simulink model "model_main4"  (R2023b)
settings: Solver=ode4  StartTime=0.0  StopTime=1000  FixedStep=dt  RelTol=1e-3
values from neighbouring files (symbols this model uses):
  dt = 0.01    [model_init.m]
  Iws = diag([1 1 1 1])*0.227    [model_init.m]
  m_tot = 3019.19    [model_init.m]
  Omega1_init = 1000*rpm2rad    (= 104.71975512)    [model_init.m]
  Omega2_init = 1000*rpm2rad    (= 104.71975512)    [model_init.m]
  Omega3_init = 1000*rpm2rad    (= 104.71975512)    [model_init.m]
  Omega4_init = 1000*rpm2rad    (= 104.71975512)    [model_init.m]
  qb0 = eul2quat(ag0','ZYX')'    [model_init.m]
  rad2rpm = 1/rpm2rad    (= 9.54929658551)    [model_init.m]
  RCS_F = 1.0    (= 1)    [model_init.m]
  RCS_Pos = [RCS1_POS , RCS2_POS , RCS3_POS , RCS4_POS ,            RCS5_POS , RCS6_POS , RCS7_POS , RCS8_POS ,            RCS9_POS , RCS10_POS, RCS11_POS, RCS12_POS,            RCS13_POS, RCS14_POS, RCS15_POS, RCS16_POS]    [model_init.m]
  RCS_PWM_Freq = 0.5    [model_init.m]
  RCS_Sampling_time = 0.01    [model_init.m]
  RCS_THR_vec = [RCS1_THR , RCS2_THR , RCS3_THR , RCS4_THR,                 RCS5_THR , RCS6_THR , RCS7_THR , RCS8_THR,                 RCS9_THR , RCS10_THR, RCS11_THR, RCS12_THR,                 RCS13_THR, RCS14_THR, RCS15_THR, RCS16_THR]    [model_init.m]
  REL_TS_POS_I_0 = TS_pos0 - SC_pos0    [model_init.m]
  REL_TS_VEL_I_0 = TS_vel0 - SC_vel0    [model_init.m]
  RW_As = [RW1_Axis,RW2_Axis,RW3_Axis,RW4_Axis]    [model_init.m]
  RW_Omegad_max = 4200*rpm2rad    (= 439.822971503)    [model_init.m]
  SC_Ib = [1257.52 -0.07285  -0.0345 ... (first row only)    [model_init.m]
  SC_state0 = kepel_statvec (SC_Kepler)    [model_init.m]
  TS_Ib = diag([1 1 1])    [model_init.m]
  TS_qb0 = angle2quat(deg2rad(0),deg2rad(0),deg2rad(0),'ZYX')'    [model_init.m]
  TS_state0 = kepel_statvec (TS_Kepler)    [model_init.m]
  TS_wb0 = deg2rad([0 0 0]')    [model_init.m]
  wb0 = [0 0 0]'    [model_init.m]
undefined symbols (not defined in the file or in its folder): norm_Ib, RCS_F_vec, RCS_pos, RW_Max_Speed, SS_Total_Mass, TC_Kepler
libraries: simulink x16, simulink_extras x13, sharedtransform x9, aerolibutil x8
(part 2 of 2)

== matlab function model_main4/Subsystem/Attitude_PD_control1 ==
  settings: updateMethod=DISCRETE
  data: F_B_cmd output; r_I input; v_I input; q_IB input; r_d input; v_d input; a_d input; m input
function F_B_cmd  = CTRL_WRENCH_6DOF(r_I, v_I, q_IB, r_d, v_d, a_d, m)
%#codegen
% ============================================================
% Controller block
% Input :
%   r_I      [3x1] current position in inertial frame
%   v_I      [3x1] current velocity in inertial frame
%   q_IB     [4x1] quaternion [qw qx qy qz], Body -> Inertial
%   omega_B  [3x1] current angular velocity in body frame
%
%   r_d      [3x1] desired position in inertial frame
%   v_d      [3x1] desired velocity in inertial frame
%   a_d      [3x1] desired acceleration in inertial frame
%   q_d      [4x1] desired quaternion, Body -> Inertial
%   omega_d_B[3x1] desired angular velocity in body frame
%
%   m        scalar mass
%   J        [3x3] inertia matrix in body frame
%
% Output:
%   F_B_cmd    [3x1] desired total body force
%   tau_B_cmd  [3x1] desired total body torque
% ============================================================

    % -------------------------
    % Quaternion normalize
    % -------------------------
    q_IB = quat_normalize(q_IB); 

    % -------------------------
    % Gains (example)
    % -------------------------
    Kp_r = 10*diag([0.01, 0.006, 0.006]);   % position gain
    Kd_r = 100*diag([0.01, 0.01, 0.01]);   % velocity damping
 
    % Kp_r = diag([0.010, 0.010, 0.010]);   % position gain
    % Kd_r = diag([0.060, 0.060, 0.060]);   % velocity damping

    % -------------------------
    % Position control
    % inertial acceleration command
    % -------------------------
    e_r = r_I - r_d;
    e_v = v_I - v_d;

    a_cmd   = a_d - Kp_r * e_r - Kd_r * e_v;
    F_I_cmd = m * a_cmd;

    % Convert inertial force -> body force
    R_IB    = quat_to_rotm(q_IB);
    F_B_cmd = R_IB.' * F_I_cmd;
 
end


% ============================================================
% Local helper functions
% ============================================================

function qn = quat_normalize(q)
    n = norm(q);
    if n < 1e-12
        qn = [1;0;0;0];
    else
        qn = q / n;
    end
end
 

function R = quat_to_rotm(q)
    % q = [qw qx qy qz], Body -> Inertial
    qw = q(1); qx = q(2); qy = q(3); qz = q(4);

    R = [1-2*(qy^2+qz^2),   2*(qx*qy-qz*qw),   2*(qx*qz+qy*qw);
         2*(qx*qy+qz*qw),   1-2*(qx^2+qz^2),   2*(qy*qz-qx*qw);
         2*(qx*qz-qy*qw),   2*(qy*qz+qx*qw),   1-2*(qx^2+qy^2)];
end

== matlab function model_main4/Subsystem/Thruster Allocation ==
  settings: updateMethod=DISCRETE
  data: u_pwm output; F_B_cmd input; tau_B_cmd input; F_B_real output; tau_B_real output; r input; d input; F_max input
function [u_pwm, F_B_real, tau_B_real] = ALLOC_THRUSTER_PWM_16(F_B_cmd, tau_B_cmd, r, d, F_max)
%#codegen
% ============================================================
% Allocation block
% Input :
%   F_B_cmd    [3x1] desired total body force
%   tau_B_cmd  [3x1] desired total body torque
%
% Output:
%   u_pwm      [12x1] thruster duty command, 0 ~ 1
%   F_B_real   [3x1] realized body force after allocation
%   tau_B_real [3x1] realized body torque after allocation
%
% Example:
%   12-thruster layout for 6DoF control
%   Replace thruster geometry / Tmax below with your real spacecraft values.
% ============================================================

    % Build 6x12 thruster mapping matrix A
    A = build_thruster_matrix( 16, r, d, F_max);

    % Desired wrench
    w_cmd = [F_B_cmd; tau_B_cmd];

    % Bounded least-squares allocation: 0 <= u <= 1
    u_pwm = bounded_allocator_0_1(A, w_cmd);

    % Realized wrench
    w_real     = A * u_pwm;
    F_B_real   = w_real(1:3);
    tau_B_real = w_real(4:6);
end


% ============================================================
% Thruster layout
% ============================================================
function A = build_thruster_matrix(N, r, d, F_max)
    % --------------------------------------------------------
    % Example spacecraft half-size [m]
    % Replace with your real geometry
    % --------------------------------------------------------
    % L = 0.50;   % lever arm

    % --------------------------------------------------------
    % Max thrust of each thruster [N]
    % Replace with your real thruster max force
    % --------------------------------------------------------
    Tmax = F_max * ones(N,1);

    % --------------------------------------------------------
    % Thruster positions r_i in body frame [m]
    % Each column is one thruster position
    % --------------------------------------------------------
    % r = [ ...
    %      0,   0,   0,   0,   L,  -L,   L,  -L,   L,  -L,   L,  -L;
    %      L,  -L,   L,  -L,   0,   0,   0,   0,   L,   L,  -L,  -L;
    %      L,  -L,  -L,   L,   L,  -L,  -L,   L,   0,   0,   0,   0 ];

    % --------------------------------------------------------
    % Thruster unit directions d_i in body frame
    %
    % T1,T2 : +X
    % T3,T4 : -X
    % T5,T6 : +Y
    % T7,T8 : -Y
    % T9,T10: +Z
    % T11,T12:-Z
    % --------------------------------------------------------
    % d = [ ...
    %      1,   1,  -1,  -1,   0,   0,   0,   0,   0,   0,   0,   0;
    %      0,   0,   0,   0,   1,   1,  -1,  -1,   0,   0,   0,   0;
    %      0,   0,   0,   0,   0,   0,   0,   0,   1,   1,  -1,  -1 ];

    % --------------------------------------------------------
    % Build A = [F; tau], size 6x12
    % --------------------------------------------------------
    A = zeros(6,N);

    for i = 1:N
        f_i       = Tmax(i) * d(:,i);
        tau_i     = cross(r(:,i), f_i);
        A(:,i)    = [f_i; tau_i];
    end
end


% ============================================================
% Bounded allocator: 0 <= u <= 1
% Codegen-friendly fixed-size active-set style
% ============================================================
function u = bounded_allocator_0_1(A, w_cmd)
    N = 16;
    u = zeros(N,1);

    % free_mask(i)=true means this thruster is still free to solve
    free_mask = true(N,1);

    lambda = 1e-8;   % small damping

    for iter = 1:(N+1)

        % Residual after fixed/saturated thrusters
        w_res = w_cmd;
        for i = 1:N
            if ~free_mask(i)
                w_res = w_res - A(:,i) * u(i);
            end
        end

        % Collect free columns into Af (fixed-size construction)
        Af  = zeros(6,N);
        idx = zeros(N,1);
        nf  = 0;

        for i = 1:N
            if free_mask(i)
                nf = nf + 1;
                idx(nf) = i;
                Af(:,nf) = A(:,i);
            end
        end

        if nf == 0
            break;
        end

        % Minimum-norm damped solution on free set
        M       = Af * Af.' + lambda * eye(6);
        uf_full = Af.' * (M \ w_res);   % size Nx1, only first nf entries used

        % Put candidate solution into u
        for k = 1:nf
            i = idx(k);
            u(i) = uf_full(k);
        end

        % Check bounds and fix saturated variables
        violated = false;
        for k = 1:nf
            i = idx(k);

            if u(i) < 0
                u(i) = 0;
                free_mask(i) = false;
                violated = true;

            elseif u(i) > 1
                u(i) = 1;
                free_mask(i) = false;
                violated = true;
            end
        end

        if ~violated
            break;
        end
    end

    % Final clipping
    for i = 1:N
        if u(i) < 0
            u(i) = 0;
        elseif u(i) > 1
            u(i) = 1;
        end
    end
end

== matlab function model_main4/saturation ==
  data: max_speed input; res output; Omega_mea input; torque_cmd input
function res  = saturation(max_speed, Omega_mea, torque_cmd)

Omega1_mea = Omega_mea(1);
Omega2_mea = Omega_mea(2);
Omega3_mea = Omega_mea(3);
Omega4_mea = Omega_mea(4);

if abs(Omega1_mea)> max_speed
    res1 = 0;
else
    res1 = torque_cmd(1);
end

if abs(Omega2_mea)>max_speed
    res2 = 0;
else
    res2 = torque_cmd(2);
end

if abs(Omega3_mea)>max_speed
    res3 = 0;
else
    res3 = torque_cmd(3);
end

if abs(Omega4_mea)>max_speed
    res4 = 0;
else
    res4 = torque_cmd(4);
end

res = [res1,res2,res3,res4]';

end

== matlab function model_main4/TS 6-DOF Dynamics ==
  data: w input; x input; Ib input; wd output; T_ext input; F_ext input; xd output
function [wd, xd]  = eq_propagate(w, x, Ib, T_ext, F_ext)
% % 
% 출력 1: 위성 동체 좌표계 각가속도
% 출력 2: 관성좌표계 선가속도

%% Rotational Motion
% wd = [0 0 0]';
wd = inv(Ib)*(T_ext - cross(w, Ib*w));

%% Translational Motion


u  = 3.9860064e+14; % earth gravitional parameter
Re = 6378137;      % earth radius [m]

xd = zeros(size(x));

v1_i = x(4); % x1 = dx/dt
v2_i = x(5); % y1 = dy/dt
v3_i = x(6); % z1 = dz/dt
p1_i = x(1); % x
p2_i = x(2); % y
p3_i = x(3); % z

r=sqrt(p1_i^2+p2_i^2+p3_i^2);

% % %   Keplar Motion Equatnion
% % %  => r_dd + u/(r^3)r_ = 0 => r_dd = -u/(r^3)r_
xd(1) = v1_i;
xd(2) = v2_i;
xd(3) = v3_i;
xd(4) = -u*p1_i/(r^3) +  F_ext(1);
xd(5) = -u*p2_i/(r^3) +  F_ext(2);
xd(6) = -u*p3_i/(r^3) +  F_ext(3);

end

== matlab function model_main4/Subsystem/Attitude_PD_control2 ==
  settings: updateMethod=DISCRETE
  data: q_err input; omega_B input; omega_d_B input; J input; tau_B_cmd output
function tau_B_cmd  = CTRL_WRENCH_6DOF(q_err, omega_B, omega_d_B, J)
%#codegen
% ============================================================
% Controller block
% Input :
%   r_I      [3x1] current position in inertial frame
%   v_I      [3x1] current velocity in inertial frame
%   q_IB     [4x1] quaternion [qw qx qy qz], Body -> Inertial
%   omega_B  [3x1] current angular velocity in body frame
%
%   r_d      [3x1] desired position in inertial frame
%   v_d      [3x1] desired velocity in inertial frame
%   a_d      [3x1] desired acceleration in inertial frame
%   q_d      [4x1] desired quaternion, Body -> Inertial
%   omega_d_B[3x1] desired angular velocity in body frame
%
%   m        scalar mass
%   J        [3x3] inertia matrix in body frame
%
% Output:
%   F_B_cmd    [3x1] desired total body force
%   tau_B_cmd  [3x1] desired total body torque
% ============================================================
 
    % -------------------------
    % Gains (example)
    % -------------------------
    Kq   = J*diag([0.3, 0.3, 0.3]);   % attitude gain
    Kw   = J*diag([5, 5, 5]);   % angular-rate damping

    % Kq   = diag([10.0, 10.0, 10.0]);   % attitude gain
    % Kw   = diag([6.0,  6.0,  6.0 ]);   % angular-rate damping
    % -------------------------
 
    % -------------------------
    % Attitude control 
    % -------------------------
 
    % shortest-path quaternion
    if q_err(1) < 0
        q_err = -q_err;
    end

    e_w = omega_B - omega_d_B;

    % PD + gyro compensation
    tau_B_cmd = -Kq * q_err(2:4) ...
                -Kw * e_w ...
                +cross(omega_B, J * omega_B);
end


% ============================================================
% Local helper functions
% ============================================================

function qn = quat_normalize(q)
    n = norm(q);
    if n < 1e-12
        qn = [1;0;0;0];
    else
        qn = q / n;
    end
end

function qc = quat_conj(q)
    qc = [q(1); -q(2); -q(3); -q(4)];
end

function q = quat_mul(q1, q2)
    % Hamilton product
    w1 = q1(1); x1 = q1(2); y1 = q1(3); z1 = q1(4);
    w2 = q2(1); x2 = q2(2); y2 = q2(3); z2 = q2(4);

    q = [ w1*w2 - x1*x2 - y1*y2 - z1*z2;
          w1*x2 + x1*w2 + y1*z2 - z1*y2;
          w1*y2 - x1*z2 + y1*w2 + z1*x2;
          w1*z2 + x1*y2 - y1*x2 + z1*w2 ];
end

== matlab function model_main4/RCS_Position&Attitude_Controller ==
  settings: updateMethod=DISCRETE
  data: r_rel input; v_rel input; r_ref input; v_ref input; a_ref input; q input; q_err input; w_err input; wb input; F_cmd_B output; tau_cmd_B output; m_sc input; Ib input; Kp_pos input; Kd_pos input; Kp_att input; Kd_att input; r_err output; v_err output; q output; q_err_vec output; w_err output; a_cmd output
function [F_cmd_B, tau_cmd_B, r_err, v_err, q, q_err_vec, w_err, a_cmd] = ...
    relative_position_los_controller( ...
    r_rel, v_rel, ...          % [3x1] relative position/velocity
    r_ref, v_ref, a_ref, ...   % [3x1] desired relative pos/vel/acc
    q, q_err, w_err, wb, m_sc, Ib, Kp_pos, Kd_pos, Kp_att, Kd_att)
%#codegen
%
% q, q_los_ref : scalar-first quaternion [qw qx qy qz]'
%                body -> reference
% r_rel, r_ref, v_rel, v_ref, a_ref : reference frame 기준
%
% 출력:
% F_cmd_B   : [3x1] body frame force command
% tau_cmd_B : [3x1] body frame torque command

F_cmd_B   = zeros(3,1);
tau_cmd_B = zeros(3,1);
r_err     = zeros(3,1);
v_err     = zeros(3,1);
q_err_vec = zeros(3,1);
% w_err     = zeros(3,1);
a_cmd     = zeros(3,1);

%% 1) Relative position controller
r_err = r_ref - r_rel;
v_err = v_ref - v_rel;

a_cmd = a_ref + Kp_pos * r_err + Kd_pos * v_err;
F_cmd_R = m_sc * a_cmd;

%% 2) Reference frame -> body frame
% q : body -> reference
% therefore F_B = C_BR' * F_R
C_BR   = quat_to_dcm_sf(q);
F_cmd_B = C_BR' * F_cmd_R;

%% 3) LOS attitude controller

% shortest path
% if q_err(1) < 0
%     q_err = -q_err;
% end

q_err_vec = q_err(2:4);

tau_cmd_B = Kp_att * q_err_vec + Kd_att * w_err + cross(wb, Ib*wb);
end


function q_out = quat_mul_sf(a, b)
% scalar-first quaternion multiplication
q_out = [ a(1)*b(1) - a(2)*b(2) - a(3)*b(3) - a(4)*b(4);
    a(1)*b(2) + a(2)*b(1) + a(3)*b(4) - a(4)*b(3);
    a(1)*b(3) - a(2)*b(4) + a(3)*b(1) + a(4)*b(2);
    a(1)*b(4) + a(2)*b(3) - a(3)*b(2) + a(4)*b(1) ];
end


function C = quat_to_dcm_sf(q)
% scalar-first quaternion, body -> reference
q = q / (sqrt(sum(q.^2)) + 1e-12);

qw = q(1);
qx = q(2);
qy = q(3);
qz = q(4);

C = [1-2*(qy*qy+qz*qz),   2*(qx*qy-qw*qz),   2*(qx*qz+qw*qy);
    2*(qx*qy+qw*qz),     1-2*(qx*qx+qz*qz), 2*(qy*qz-qw*qx);
    2*(qx*qz-qw*qy),     2*(qy*qz+qw*qx),   1-2*(qx*qx+qy*qy)];
end

== matlab function model_main4/RCS_Relative_Position_Control_Allocation2 ==
  settings: updateMethod=DISCRETE
  data: F_cmd input; tau_cmd input; RCS_pos input; RCS_F_vec input; Tmax input; duty output; F_est output; tau_est output; F_err output; tau_err output; sat_ratio output; wF input; wT input
function [duty, F_est, tau_est, F_err, tau_err, sat_ratio] = ...
    rcs_force_torque_allocator(F_cmd, tau_cmd, RCS_pos, RCS_F_vec, Tmax, wF, wT)
%#codegen
%
% F_cmd      : [3x1] commanded force in body frame [N]
% tau_cmd    : [3x1] commanded torque in body frame [N*m]
% RCS_pos    : [3xN] thruster positions in body frame [m]
% RCS_F_vec  : [3xN] thruster direction vectors
% Tmax       : scalar, max thrust of one thruster [N]
% wF         : scalar, force tracking weight
% wT         : scalar, torque tracking weight
%
% duty       : [N x 1], 0~1
% F_est      : [3x1], achieved force [N]
% tau_est    : [3x1], achieved torque [N*m]
% F_err      : [3x1], force error [N]
% tau_err    : [3x1], torque error [N*m]
% sat_ratio  : saturated thruster ratio

    N = size(RCS_pos, 2);

    duty      = zeros(N,1);
    F_est     = zeros(3,1);
    tau_est   = zeros(3,1);
    F_err     = zeros(3,1);
    tau_err   = zeros(3,1);
    sat_ratio = 0;

    Fmat = zeros(3, N);
    Tmat = zeros(3, N);

    for i = 1:N
        dir_i = RCS_F_vec(:,i);
        nrm   = sqrt(sum(dir_i.^2));

        if nrm > 1e-12
            dir_i = dir_i / nrm;
        else
            dir_i = [0;0;0];
        end

        Fi = Tmax * dir_i;
        Ti = cross3(RCS_pos(:,i), Fi);

        Fmat(:,i) = Fi;
        Tmat(:,i) = Ti;
    end

    % Solve:
    % min || wF*(Fmat*u - F_cmd) ||^2 + || wT*(Tmat*u - tau_cmd) ||^2
    % s.t. 0 <= u <= 1

    A = [wF * Fmat;
         wT * Tmat];

    b = [wF * F_cmd;
         wT * tau_cmd];

    H = A' * A + 1e-8 * eye(N);
    g = A' * b;

    alpha = 1.0 / (trace(H) + 1e-9);
    u = zeros(N,1);

    for k = 1:150
        grad = H * u - g;
        u    = u - alpha * grad;

        for j = 1:N
            if u(j) < 0
                u(j) = 0;
            elseif u(j) > 1
                u(j) = 1;
            end
        end
    end

    duty    = u;
    F_est   = Fmat * duty;
    tau_est = Tmat * duty;

    F_err   = F_cmd   - F_est;
    tau_err = tau_cmd - tau_est;

    sat_ratio = sum(duty > 0.999) / N;
end


function c = cross3(a, b)
    c = [ a(2)*b(3) - a(3)*b(2);
          a(3)*b(1) - a(1)*b(3);
          a(1)*b(2) - a(2)*b(1) ];
end

== matlab function model_main4/Mission_Supporter ==
  settings: updateMethod=DISCRETE
  data: flag output; res_pos input; stop output
function [flag, stop]  = Mission_Supporter(res_pos)

d_norm = norm(res_pos);
d_parking = 5;

if abs((d_norm - d_parking)) > 1 
    flag = 0; % approach, RCS on

else
    flag = 1; % station keeping, RW on
    
end

if d_norm <= 0.1
    stop = 1;
else 
    stop = 0;
end

== matlab function model_main4/command_generator ==
  settings: updateMethod=DISCRETE
  data: rel_p_cmd output; flag input; rel_v_cmd output; Kp_pos output; Kd_pos output
function [rel_p_cmd,rel_v_cmd,Kp_pos,Kd_pos]  = Mission_Supporter(flag)

if flag == 0
    rel_p_cmd = [5 0 0]';
    rel_v_cmd = [0 0 0]';
    Kp_pos = 0.3;
    Kd_pos = 17;    
else
    rel_p_cmd = [5 0 0]';
    rel_v_cmd = [0 0 0]';
    Kp_pos =   0.3;
    Kd_pos = 17.0;    
end


end

== matlab function model_main4/Get LOS Quaternion ==
  data: r_rel input; q output; ang_deg output; axis_rot output
function [q, ang_deg, axis_rot] = boresight_to_target_quat(r_rel)
%#codegen
% ============================================================
% boresight_to_target_quat
%
% Input:
%   r_rel    [3x1] : relative position vector
%
% Output:
%   q        [4x1] : quaternion [w; x; y; z]
%                    rotating boresight [1;0;0] to r_rel direction
%   ang_deg  [1x1] : rotation angle in degrees
%   axis_rot [3x1] : rotation axis (unit vector)
%
% Notes:
%   - boresight reference is fixed as [1; 0; 0]
%   - quaternion is scalar-first
%   - handles parallel / anti-parallel edge cases
% ============================================================

    % Reference boresight
    b_ref = [1; 0; 0];

    % Small threshold
    eps_val = 1e-12;

    % Check input norm
    r_norm = norm(r_rel);
    if r_norm < eps_val
        % Undefined direction
        q = [1; 0; 0; 0];
        ang_deg = 0;
        axis_rot = [1; 0; 0];
        return;
    end

    % Normalize target direction
    v = r_rel / r_norm;
    u = b_ref;

    % Dot product
    c = dot(u, v);
    c = max(min(c, 1.0), -1.0);   % numerical safety

    % Case 1: same direction
    if c > 1 - 1e-10
        q = [1; 0; 0; 0];
        ang_deg = 0;
        axis_rot = [1; 0; 0];
        return;
    end

    % Case 2: opposite direction
    if c < -1 + 1e-10
        % Need 180 deg rotation about any axis orthogonal to [1;0;0]
        % Choose y-axis
        axis_rot = [0; 1; 0];
        q = [0; axis_rot];   % cos(pi/2)=0, sin(pi/2)=1
        ang_deg = 180;
        return;
    end

    % General case
    cross_uv = cross(u, v);

    % Robust quaternion from two vectors:
    % q = [1 + dot(u,v); cross(u,v)] then normalize
    q = [1 + c;
         cross_uv(1);
         cross_uv(2);
         cross_uv(3)];

    q = q / norm(q);

    % Rotation angle
    ang_rad = 2 * acos(q(1));
    ang_deg = ang_rad * 180 / pi;

    % Rotation axis
    s = sqrt(1 - q(1)^2);
    if s < 1e-10
        axis_rot = [1; 0; 0];
    else
        axis_rot = q(2:4) / s;
    end
end

== matlab function model_main4/Subsystem/Attitude_PD_control ==
  settings: updateMethod=DISCRETE
  data: u_torq output; q_err input; w_err input
function u_torq = att_pd_control(q_err, w_err)

persistent first_flg
persistent I_save

dt = 0.01;

if isempty(first_flg)
    first_flg = 1;
    I_save = [0 0 0]';
end

K1 = 10.1*diag([1 1 1]);
K2 = 8.2*diag([1 1 1]);
K3 = 0.1*diag([1 1 1]);

q_err_ = [q_err(2), q_err(3), q_err(4)]';

u_torq = K1*q_err_ + K2*w_err + K3*I_save;

I_save = I_save + q_err_ * dt;

end

== matlab function model_main4/Subsystem/THR_Allocation ==
  data: pwm output; tau_cmd input; F_on input; f input; r_thr input
function pwm = RCS_Torque2PWM(tau_cmd, F_on, f, r_thr)
%#codegen
% ============================================================
% Minimal RCS allocation: torque command -> PWM duty (0..1)
%   tau ≈ sum_i r_i x (f_i * F_on_i * pwm_i)
%
% Inputs:
%   tau_cmd [3x1]
%   F_on    scalar or [12x1]
%   f       [3x12]  (columns are unit vectors)
%   r_thr   [3x12]  (columns are position vectors wrt CoM)
%
% Output:
%   pwm     [12x1] duty in [0,1]
% ============================================================
N = 16;
% F_on -> 12x1
if isscalar(F_on)
    Fon = F_on * ones(N,1);
else
    Fon = F_on(:);
end

% Build effectiveness matrix B (3x12): tau = B * pwm
B = zeros(3,N);
for i = 1:N
    Fi = Fon(i);
    B(:,i) = cross3(r_thr(:,i), f(:,i) * Fi);  % torque from pwm=1
end

% Unconstrained least-squares solution (minimum-norm)
pwm = B' * ((B*B') \ tau_cmd);

% Clamp to [0,1]
for i=1:N
    if pwm(i) < 0, pwm(i) = 0; end
    if pwm(i) > 1, pwm(i) = 1; end
end

end

function c = cross3(a,b)
c = [ a(2)*b(3) - a(3)*b(2);
      a(3)*b(1) - a(1)*b(3);
      a(1)*b(2) - a(2)*b(1) ];
end

== matlab function model_main4/Quaternion_Kinematics ==
  data: w input; qd output; q input
function qd = fcn(w,q)

F_q = (1/2)*[0 -w(1) -w(2) -w(3);
       w(1) 0 w(3) -w(2);
       w(2) -w(3) 0 w(1);
       w(3) w(2) -w(1) 0];

qd = F_q*q;

end

== matlab function model_main4/Enabled Subsystem/QP Opt ==
  settings: updateMethod=DISCRETE
  data: tau_des input; u_rw_cmd output; Omega_rw input; dt input; tau_body_cmd output; exitflag_out output; RW_max_speed input
function [u_rw_cmd, tau_body_cmd, exitflag_out] = RW4_QP_Controller(tau_des, Omega_rw, dt, RW_max_speed)
%#codegen
%
% 4-wheel Reaction Wheel QP controller
% tau_body = -A_rw * u_rw
%
% Inputs:
%   tau_des   [3x1] desired body torque
%   Omega_rw  [4x1] current wheel speeds [rad/s]
%   u_prev    [4x1] previous wheel torque command [N*m]
%   dt        scalar control period [s]
%
% Outputs:
%   u_rw_cmd     [4x1] wheel motor torque command
%   tau_body_cmd [3x1] actual body torque from RW
%   exitflag_out scalar

persistent u_save;

if isempty(u_save)
    u_save = [0 0 0 0]';
end

u_rw_cmd     = zeros(4,1);
tau_body_cmd = zeros(3,1);
exitflag_out = 0;

tau_des  = reshape(tau_des,  [3,1]);
Omega_rw = reshape(Omega_rw, [4,1]);
u_prev   = u_save;

% =========================
% RW axis matrix (3x4)
% =========================
A_rw = [ 0.70710678,  0.0,        -0.70710678,  0.0;
         0.0,         0.70710678,  0.0,        -0.70710678;
         0.70710678,  0.70710678,  0.70710678,  0.70710678 ];

% =========================
% User parameters
% =========================
% Torque tracking weight (body torque tracking)
Wtau = diag([10.0, 10.0, 10.0]);

% Wheel torque magnitude penalty
Wu = 1e-3 * eye(4);

% Wheel torque smoothing penalty
Wr = 1e-2 * eye(4);

% Optional wheel-speed centering penalty
% Start with very small values. Increase later if wheel speeds drift too much.
Wh = zeros(4,4);
% 예: Wh = 1e-6 * eye(4);

% Wheel inertia about spin axis [kg*m^2]
Jw = 0.227*[1;1;1;1];

% Wheel torque limits [N*m]
u_max = [0.2; 0.2; 0.2; 0.2];
u_min = -u_max;

% Wheel torque rate limits [N*m/s]
du_max = [0.20; 0.20; 0.20; 0.20];
du_min = -du_max;

% Wheel speed limits [rad/s]
Omega_max = [RW_max_speed;RW_max_speed;RW_max_speed;RW_max_speed];
Omega_min = -Omega_max;

% =========================
% QP construction
%
% minimize 0.5*|| -A_rw*u - tau_des ||^2_Wtau
%        + 0.5*u'*Wu*u
%        + 0.5*(u-u_prev)'*Wr*(u-u_prev)
%        + 0.5*(Omega_next)'*Wh*(Omega_next)
%
% Omega_next = Omega_rw + D*u
% D = diag(dt./Jw)
% =========================

D = diag(dt ./ Jw);

H = A_rw' * Wtau * A_rw + Wu + Wr + D' * Wh * D;
f = A_rw' * Wtau * tau_des - Wr * u_prev + D' * Wh * Omega_rw;

% Make H numerically symmetric
H = 0.5 * (H + H');

% =========================
% Constraints
% 1) wheel torque bounds
% 2) wheel torque rate bounds
% 3) next-step wheel speed bounds
% =========================

% Torque-rate bounds
lb_rate = u_prev + du_min * dt;
ub_rate = u_prev + du_max * dt;

% Speed-next bounds
% Omega_next = Omega_rw + dt*(u./Jw)
% => u >= Jw .* (Omega_min - Omega_rw)/dt
% => u <= Jw .* (Omega_max - Omega_rw)/dt
lb_speed = Jw .* ((Omega_min - Omega_rw) / dt);
ub_speed = Jw .* ((Omega_max - Omega_rw) / dt);

% Final bounds
lb = max(u_min, max(lb_rate, lb_speed));
ub = min(u_max, min(ub_rate, ub_speed));

% Feasibility repair
for i = 1:4
    if lb(i) > ub(i)
        c = 0.5 * (lb(i) + ub(i));
        lb(i) = c;
        ub(i) = c;
    end
end

% Empty linear inequality/equality constraints
A   = zeros(0,4);
b   = zeros(0,1);
Aeq = zeros(0,4);
beq = zeros(0,1);

% Initial guess for active-set
x0 = min(max(u_prev, lb), ub);

% quadprog codegen-friendly option
options = optimoptions('quadprog', ...
    'Algorithm', 'active-set', ...
    'ConstraintTolerance', 1e-6, ...
    'OptimalityTolerance', 1e-6, ...
    'StepTolerance', 1e-12, ...
    'MaxIterations', 50);

[u_sol, ~, exitflag] = quadprog(H, f, A, b, Aeq, beq, lb, ub, x0, options);

if exitflag <= 0 || isempty(u_sol)
    u_rw_cmd = x0;
else
    u_rw_cmd = u_sol;
end

tau_body_cmd = -A_rw * u_rw_cmd;
u_save = u_rw_cmd;
exitflag_out = exitflag;

== matlab function model_main4/Subsystem/Get LOS Quaternion7 ==
  settings: updateMethod=DISCRETE
  data: r_rel input; v_rel input; r_ref input; v_ref input; a_ref input; q input; q_err input; w_err input; F_cmd_B output; tau_cmd_B output; m_sc input; Kp_pos input; Kd_pos input; Kp_att input; Kd_att input; r_err output; v_err output; q output; q_err_vec output; w_err output; a_cmd output
function [F_cmd_B, tau_cmd_B, r_err, v_err, q, q_err_vec, w_err, a_cmd] = ...
    relative_position_los_controller( ...
    r_rel, v_rel, ...          % [3x1] relative position/velocity
    r_ref, v_ref, a_ref, ...   % [3x1] desired relative pos/vel/acc
    q, q_err, w_err, ...                  % [4x1], [3x1] current attitude/angular velocity
    m_sc, Kp_pos, Kd_pos, Kp_att, Kd_att)
%#codegen
%
% q, q_los_ref : scalar-first quaternion [qw qx qy qz]'
%                body -> reference
% r_rel, r_ref, v_rel, v_ref, a_ref : reference frame 기준
%
% 출력:
% F_cmd_B   : [3x1] body frame force command
% tau_cmd_B : [3x1] body frame torque command

    F_cmd_B   = zeros(3,1);
    tau_cmd_B = zeros(3,1);
    r_err     = zeros(3,1);
    v_err     = zeros(3,1);
    q_err_vec = zeros(3,1);
    % w_err     = zeros(3,1);
    a_cmd     = zeros(3,1);

    %% 1) Relative position controller
    r_err = r_ref - r_rel;
    v_err = v_ref - v_rel;

    a_cmd = a_ref + Kp_pos * r_err + Kd_pos * v_err;
    F_cmd_R = m_sc * a_cmd;

    %% 2) Reference frame -> body frame
    % q : body -> reference
    % therefore F_B = C_BR' * F_R
    C_BR   = quat_to_dcm_sf(q);
    F_cmd_B = C_BR' * F_cmd_R;

    %% 3) LOS attitude controller

    % shortest path
    if q_err(1) < 0
        q_err = -q_err;
    end

    q_err_vec = q_err(2:4);

    tau_cmd_B = Kp_att * q_err_vec + Kd_att * w_err;
end


function q_out = quat_mul_sf(a, b)
% scalar-first quaternion multiplication
    q_out = [ a(1)*b(1) - a(2)*b(2) - a(3)*b(3) - a(4)*b(4);
              a(1)*b(2) + a(2)*b(1) + a(3)*b(4) - a(4)*b(3);
              a(1)*b(3) - a(2)*b(4) + a(3)*b(1) + a(4)*b(2);
              a(1)*b(4) + a(2)*b(3) - a(3)*b(2) + a(4)*b(1) ];
end


function C = quat_to_dcm_sf(q)
% scalar-first quaternion, body -> reference
    q = q / (sqrt(sum(q.^2)) + 1e-12);

    qw = q(1);
    qx = q(2);
    qy = q(3);
    qz = q(4);

    C = [1-2*(qy*qy+qz*qz),   2*(qx*qy-qw*qz),   2*(qx*qz+qw*qy);
         2*(qx*qy+qw*qz),     1-2*(qx*qx+qz*qz), 2*(qy*qz-qw*qx);
         2*(qx*qz-qw*qy),     2*(qy*qz+qw*qx),   1-2*(qx*qx+qy*qy)];
end

== matlab function model_main4/Subsystem/Subsystem1/MinOnTime_Enforcer1 ==
  settings: updateMethod=DISCRETE
  data: relay_raw input; F_gated output; t input
function F_gated = fcn(relay_raw, t)
%#codegen
% 최소 ON 시간 강제기 (MIB 기반)
% t_min_on = 0.0700 s (70 ms)
persistent t_on_start was_on;
if isempty(was_on)
    was_on     = false;
    t_on_start = 0;
end
t_min_on = 0.0700;
if relay_raw == 1 && ~was_on
    t_on_start = t;
end
if relay_raw == 1
    F_gated = 1;
elseif was_on && (t - t_on_start) < t_min_on
    F_gated = 1;   % 아직 70ms 안 됐으면 강제 ON 유지
else
    F_gated = 0;
end
was_on = (F_gated == 1);

end

== matlab function model_main4/Subsystem/Subsystem2/MinOnTime_Enforcer1 ==
  settings: updateMethod=DISCRETE
  data: relay_raw input; F_gated output; t input
function F_gated = fcn(relay_raw, t)
%#codegen
% 최소 ON 시간 강제기 (MIB 기반)
% t_min_on = 0.0700 s (70 ms)
persistent t_on_start was_on;
if isempty(was_on)
    was_on     = false;
    t_on_start = 0;
end
t_min_on = 0.0700;
if relay_raw == 1 && ~was_on
    t_on_start = t;
end
if relay_raw == 1
    F_gated = 1;
elseif was_on && (t - t_on_start) < t_min_on
    F_gated = 1;   % 아직 70ms 안 됐으면 강제 ON 유지
else
    F_gated = 0;
end
was_on = (F_gated == 1);

end

== matlab function model_main4/Subsystem/Subsystem3/MinOnTime_Enforcer1 ==
  settings: updateMethod=DISCRETE
  data: relay_raw input; F_gated output; t input
function F_gated = fcn(relay_raw, t)
%#codegen
% 최소 ON 시간 강제기 (MIB 기반)
% t_min_on = 0.0700 s (70 ms)
persistent t_on_start was_on;
if isempty(was_on)
    was_on     = false;
    t_on_start = 0;
end
t_min_on = 0.0700;
if relay_raw == 1 && ~was_on
    t_on_start = t;
end
if relay_raw == 1
    F_gated = 1;
elseif was_on && (t - t_on_start) < t_min_on
    F_gated = 1;   % 아직 70ms 안 됐으면 강제 ON 유지
else
    F_gated = 0;
end
was_on = (F_gated == 1);

end

== matlab function model_main4/Subsystem/Subsystem4/MinOnTime_Enforcer1 ==
  settings: updateMethod=DISCRETE
  data: relay_raw input; F_gated output; t input
function F_gated = fcn(relay_raw, t)
%#codegen
% 최소 ON 시간 강제기 (MIB 기반)
% t_min_on = 0.0700 s (70 ms)
persistent t_on_start was_on;
if isempty(was_on)
    was_on     = false;
    t_on_start = 0;
end
t_min_on = 0.0700;
if relay_raw == 1 && ~was_on
    t_on_start = t;
end
if relay_raw == 1
    F_gated = 1;
elseif was_on && (t - t_on_start) < t_min_on
    F_gated = 1;   % 아직 70ms 안 됐으면 강제 ON 유지
else
    F_gated = 0;
end
was_on = (F_gated == 1);

end

== matlab function model_main4/Subsystem/Subsystem5/MinOnTime_Enforcer1 ==
  settings: updateMethod=DISCRETE
  data: relay_raw input; F_gated output; t input
function F_gated = fcn(relay_raw, t)
%#codegen
% 최소 ON 시간 강제기 (MIB 기반)
% t_min_on = 0.0700 s (70 ms)
persistent t_on_start was_on;
if isempty(was_on)
    was_on     = false;
    t_on_start = 0;
end
t_min_on = 0.0700;
if relay_raw == 1 && ~was_on
    t_on_start = t;
end
if relay_raw == 1
    F_gated = 1;
elseif was_on && (t - t_on_start) < t_min_on
    F_gated = 1;   % 아직 70ms 안 됐으면 강제 ON 유지
else
    F_gated = 0;
end
was_on = (F_gated == 1);

end

== matlab function model_main4/Subsystem/Subsystem6/MinOnTime_Enforcer1 ==
  settings: updateMethod=DISCRETE
  data: relay_raw input; F_gated output; t input
function F_gated = fcn(relay_raw, t)
%#codegen
% 최소 ON 시간 강제기 (MIB 기반)
% t_min_on = 0.0700 s (70 ms)
persistent t_on_start was_on;
if isempty(was_on)
    was_on     = false;
    t_on_start = 0;
end
t_min_on = 0.0700;
if relay_raw == 1 && ~was_on
    t_on_start = t;
end
if relay_raw == 1
    F_gated = 1;
elseif was_on && (t - t_on_start) < t_min_on
    F_gated = 1;   % 아직 70ms 안 됐으면 강제 ON 유지
else
    F_gated = 0;
end
was_on = (F_gated == 1);

end

== matlab function model_main4/Subsystem/Subsystem7/MinOnTime_Enforcer1 ==
  settings: updateMethod=DISCRETE
  data: relay_raw input; F_gated output; t input
function F_gated = fcn(relay_raw, t)
%#codegen
% 최소 ON 시간 강제기 (MIB 기반)
% t_min_on = 0.0700 s (70 ms)
persistent t_on_start was_on;
if isempty(was_on)
    was_on     = false;
    t_on_start = 0;
end
t_min_on = 0.0700;
if relay_raw == 1 && ~was_on
    t_on_start = t;
end
if relay_raw == 1
    F_gated = 1;
elseif was_on && (t - t_on_start) < t_min_on
    F_gated = 1;   % 아직 70ms 안 됐으면 강제 ON 유지
else
    F_gated = 0;
end
was_on = (F_gated == 1);

end

== matlab function model_main4/Subsystem/Subsystem8/MinOnTime_Enforcer1 ==
  settings: updateMethod=DISCRETE
  data: relay_raw input; F_gated output; t input
function F_gated = fcn(relay_raw, t)
%#codegen
% 최소 ON 시간 강제기 (MIB 기반)
% t_min_on = 0.0700 s (70 ms)
persistent t_on_start was_on;
if isempty(was_on)
    was_on     = false;
    t_on_start = 0;
end
t_min_on = 0.0700;
if relay_raw == 1 && ~was_on
    t_on_start = t;
end
if relay_raw == 1
    F_gated = 1;
elseif was_on && (t - t_on_start) < t_min_on
    F_gated = 1;   % 아직 70ms 안 됐으면 강제 ON 유지
else
    F_gated = 0;
end
was_on = (F_gated == 1);

end

== matlab function model_main4/Subsystem/RCS_Relative_Position_Control_Allocation1 ==
  settings: updateMethod=DISCRETE
  data: F_cmd input; tau_cmd input; RCS_pos input; RCS_F_vec input; Tmax input; duty output; F_est output; tau_est output; F_err output; tau_err output; sat_ratio output; wF input; wT input
function [duty, F_est, tau_est, F_err, tau_err, sat_ratio] = ...
    rcs_force_torque_allocator(F_cmd, tau_cmd, RCS_pos, RCS_F_vec, Tmax, wF, wT)
%#codegen
%
% F_cmd      : [3x1] commanded force in body frame [N]
% tau_cmd    : [3x1] commanded torque in body frame [N*m]
% RCS_pos    : [3xN] thruster positions in body frame [m]
% RCS_F_vec  : [3xN] thruster direction vectors
% Tmax       : scalar, max thrust of one thruster [N]
% wF         : scalar, force tracking weight
% wT         : scalar, torque tracking weight
%
% duty       : [N x 1], 0~1
% F_est      : [3x1], achieved force [N]
% tau_est    : [3x1], achieved torque [N*m]
% F_err      : [3x1], force error [N]
% tau_err    : [3x1], torque error [N*m]
% sat_ratio  : saturated thruster ratio

    N = size(RCS_pos, 2);

    duty      = zeros(N,1);
    F_est     = zeros(3,1);
    tau_est   = zeros(3,1);
    F_err     = zeros(3,1);
    tau_err   = zeros(3,1);
    sat_ratio = 0;

    Fmat = zeros(3, N);
    Tmat = zeros(3, N);

    for i = 1:N
        dir_i = RCS_F_vec(:,i);
        nrm   = sqrt(sum(dir_i.^2));

        if nrm > 1e-12
            dir_i = dir_i / nrm;
        else
            dir_i = [0;0;0];
        end

        Fi = Tmax * dir_i;
        Ti = cross3(RCS_pos(:,i), Fi);

        Fmat(:,i) = Fi;
        Tmat(:,i) = Ti;
    end

    % Solve:
    % min || wF*(Fmat*u - F_cmd) ||^2 + || wT*(Tmat*u - tau_cmd) ||^2
    % s.t. 0 <= u <= 1

    A = [wF * Fmat;
         wT * Tmat];

    b = [wF * F_cmd;
         wT * tau_cmd];

    H = A' * A + 1e-8 * eye(N);
    g = A' * b;

    alpha = 1.0 / (trace(H) + 1e-9);
    u = zeros(N,1);

    for k = 1:150
        grad = H * u - g;
        u    = u - alpha * grad;

        for j = 1:N
            if u(j) < 0
                u(j) = 0;
            elseif u(j) > 1
                u(j) = 1;
            end
        end
    end

    duty    = u;
    F_est   = Fmat * duty;
    tau_est = Tmat * duty;

    F_err   = F_cmd   - F_est;
    tau_err = tau_cmd - tau_est;

    sat_ratio = sum(duty > 0.999) / N;
end


function c = cross3(a, b)
    c = [ a(2)*b(3) - a(3)*b(2);
          a(3)*b(1) - a(1)*b(3);
          a(1)*b(2) - a(2)*b(1) ];
end

== matlab function model_main4/SS Attitude Control wrt ECI ==
  settings: updateMethod=DISCRETE
  data: q_err input; RW_cmd output; w_err input; As input; Kp_rw input; Kd_rw input; Ki_rw input
function RW_cmd  = Att_PD_Control(q_err, w_err, As,Kp_rw,Kd_rw,Ki_rw)

persistent I_save
persistent flg

if isempty(flg)
    flg = 1;
    I_save = [0 0 0]';
end
 
% K3 = 0.025*diag([1 1 1]);

q_e_v = [q_err(2), q_err(3), q_err(4)]';

u = Kp_rw*q_e_v + Kd_rw*w_err + Ki_rw*I_save;

RW_cmd = pinv(As)*-u;

I_save = I_save + (q_e_v*0.01);

end

== matlab function model_main4/Subsystem/MATLAB Function1 ==
  data: kepel input; statvec output
function statvec  = kepel_statvec (kepel)
%  [statvec] = kepel_statvec (kepel)
%	The function kepel_statvec transforms the keplerian
%	elements kepel into the corresponding state vector in
%	the same reference system.
%
% Input:
%	kepel
% 		vector containing the keplerian elements:
%		(1) - semimajor axis of the orbit in meters.
%		(2) - eccentricity.
%		(3) - inclinatsion in radians.
%		(4) - right ascension of ascending node in radians.
%		(5) - argument of perigee in radians.
%		(6) - mean anomaly in radians.
% Output:
%	statvec
%  		state vector in meters and meters/second.
%
% Authors:
%	Helio K. Kuga;
%	Valder M. Medeiros;
%	Valdemir Carrara		february/80		version 1.0
%	Valdemir Carrara		july 2005		(C version)
%   Valdemir Carrara            March/09        Matlab

EARTH_GRAVITY	= 3.9860064e+14;		% Earth's gravitational constant (m**3/s**2)

a    = kepel(1);	% semi-major axis
exc  = kepel(2);	% eccentricity

c1   = sqrt(1. - exc*exc);

%     rotation matrix

orb2iner = rotmaz(-kepel(4))*rotmax(-kepel(3))*rotmaz(-kepel(5));

%     Kepler's equation

E    = kepler(kepel(6), exc);

sE   = sin(E);
cE   = cos(E);
c3   = sqrt(EARTH_GRAVITY/a)/(1. - exc*cE);

%     state vector

statvec = [[a*(cE - exc), a*c1*sE, 0]*orb2iner', [-c3*sE, c1*c3*cE, 0]*orb2iner'];

end

function [rot_mat] = rotmax (angle)
% [rot_mat] = rotmax (angle)
%   To obtain the rotation matrix around the X axis given the
%   rotation angle.
% inputs:
%   angle
%       rotation angle, in radians.
% outputs:
%   rot_mat
%       rotation matrix (3, 3)
%

% Valdemir Carrara, Sep, 1998

coan    =  cos(angle);
sian    =  sin(angle);

rot_mat =  [1, 0, 0; 0, coan, sian; 0, -sian, coan];

end

function [rot_mat] = rotmay (angle)
% [rot_mat] = rotmay (angle)
%   To obtain the rotation matrix around the Y axis given the
%   rotation angle.
% inputs:
%   angle
%       rotation angle, in radians.
% outputs:
%   rot_mat
%       rotation matrix (3, 3)
%

% Valdemir Carrara, Sep, 1998


coan    =  cos(angle);
sian    =  sin(angle);

rot_mat =  [coan, 0, -sian; 0, 1, 0; sian, 0, coan];

end

function [rot_mat] = rotmaz (angle)
% [rot_mat] = rotmaz (angle)
%   To obtain the rotation matrix around the Z axis given the
%   rotation angle.
% inputs:
%   angle
%       rotation angle, in radians.
% outputs:
%   rot_mat
%       rotation matrix (3, 3)
%

% Valdemir Carrara, Sep, 1998

coan    =  cos(angle);
sian    =  sin(angle);

rot_mat =  [coan, sian, 0; -sian, coan, 0; 0, 0, 1];
end

function [eccentric] = kepler (mean_anomaly, eccentricity)
% [eccentric] = kepler (mean_anomaly, eccentricity)
%	The subroutine kepler finds a solution to the
%	kepler's equation.
%
% Input:
%	mean_anomaly
%		mean anomaly in radians.
%	eccentricity
%		eccentricity.
%
% Output:
%	eccentric
%		eccentric anomaly in radians.
%
% Authors:
%	Valder M. de Medeiros		june/81		version 2.0
%	Valdemir Carrara			july 2005	(C version)
%   Valdemir Carrara            March/09        Matlab

exc2    = eccentricity*eccentricity;
am1     = mod (mean_anomaly, 2*pi);
am2     = am1 + am1;
am3     = am1 + am2;
shoot   = am1 + eccentricity*(1. - 0.125*exc2)*sin(am1) + ...
		0.5*exc2*(sin(am2) + 0.75*eccentricity*sin(am3));
shoot   = mod (shoot, 2*pi);

e1      = 1.0;
ic      = 0;

while ((abs(e1) > 1.e-12) && (ic <= 10)) 
	e1    = (shoot - am1 - eccentricity*sin(shoot)) / ...
			(1.0 - eccentricity*cos(shoot));
    shoot = shoot - e1;
    ic    = ic + 1;
end

if (ic >= 10)
    disp ('warning ** subroutine kepler did not converge in 10 iterations');
end

eccentric = shoot;


end

== matlab function model_main4/Subsystem/TC Kepler Propagate ==
  data: initial_condition input; dfdt output; F_eci input
function dfdt  = eq_propagate(initial_condition, F_eci)
% Lectures_TwoBodyProblem.pdf
% 우주시스템입문 - 도미타 노부유키 eq(7.8) p136
% https://en.wikipedia.org/wiki/Standard_gravitational_parameter
u  = 3.9860064e+14; % earth gravitional parameter
Re = 6378137;      % earth radius [m]

dfdt = zeros(size(initial_condition));

% x=x
% x1=dx/dt
% dx1/dt = d^2(x)/dt

x1 = initial_condition(4); % x1 = dx/dt
y1 = initial_condition(5); % y1 = dy/dt
z1 = initial_condition(6); % z1 = dz/dt
x  = initial_condition(1); % x
y  = initial_condition(2); % y
z  = initial_condition(3); % z

r=sqrt(x^2+y^2+z^2);

% % %   Keplar Motion Equatnion
% % %  => r_dd + u/(r^3)r_ = 0 => r_dd = -u/(r^3)r_
dfdt(1) = x1;
dfdt(2) = y1;
dfdt(3) = z1;
dfdt(4) = -u*x/(r^3) + F_eci(1);
dfdt(5) = -u*y/(r^3) + F_eci(2);
dfdt(6) = -u*z/(r^3) + F_eci(3);

end

== matlab function model_main4/SC 6-DOF Dynamics ==
  data: w input; x input; Ib input; m_tot input; Iws input; As input; Omega input; Omegad input; RCS_mea input; RCS_pos input; RCS_vec input; wd output; R_Ib input; T_ext input; F_ext input; xd output
function [wd, xd]  = eq_propagate(w, x, Ib, m_tot, ...
                                   Iws, As, Omega, Omegad, ...
                                   RCS_mea, RCS_pos, RCS_vec, R_Ib, ...
                                   T_ext, F_ext)
% % 
% 출력 1: 위성 동체 좌표계 각가속도
% 출력 2: 관성좌표계 선가속도

% % 
RW_h = As*Iws*Omega;
RW_hd = As*Iws*Omegad;

% % 
N = 16;
RCS_f = zeros(3,N);
RCS_t = zeros(3,N);

for i = 1:N
    r_i = RCS_pos(:,i);   % position of thruster i
    d_i = RCS_vec(:,i);   % thrust direction of thruster i

    % force contribution
    RCS_f(:,i) = d_i;

    % torque contribution
    RCS_t(:,i) = cross(r_i, d_i);
end
RCS_f_total = RCS_f * RCS_mea;  % [3x1]
RCS_t_total = RCS_t * RCS_mea;  % [3x1]


%% Rotational Motion
wd = [0 0 0]';
wd = inv(Ib)*(T_ext + RCS_t_total - RW_hd - cross(w, Ib*w + RW_h));

%% Translational Motion

F_I = R_Ib * RCS_f_total;

u  = 3.9860064e+14; % earth gravitional parameter
Re = 6378137;      % earth radius [m]

xd = zeros(size(x));

v1_i = x(4); % x1 = dx/dt
v2_i = x(5); % y1 = dy/dt
v3_i = x(6); % z1 = dz/dt
p1_i = x(1); % x
p2_i = x(2); % y
p3_i = x(3); % z

r=sqrt(p1_i^2+p2_i^2+p3_i^2);

% % %   Keplar Motion Equatnion
% % %  => r_dd + u/(r^3)r_ = 0 => r_dd = -u/(r^3)r_
xd(1) = v1_i;
xd(2) = v2_i;
xd(3) = v3_i;
xd(4) = -u*p1_i/(r^3) + F_I(1)/m_tot + F_ext(1)/m_tot;
xd(5) = -u*p2_i/(r^3) + F_I(2)/m_tot + F_ext(2)/m_tot;
xd(6) = -u*p3_i/(r^3) + F_I(3)/m_tot + F_ext(3)/m_tot;

end

== matlab function model_main4/Quaternion_Kinematics1 ==
  data: w input; qd output; q input
function qd = fcn(w,q)

F_q = (1/2)*[0 -w(1) -w(2) -w(3);
       w(1) 0 w(3) -w(2);
       w(2) -w(3) 0 w(1);
       w(3) w(2) -w(1) 0];

qd = F_q*q;

end
